simulink model "ASM_Traffic_V2X_Complete_Model_2"  (R2019a)
settings: Solver=ode1  StartTime=SIM.tstart.v  StopTime=Inf  FixedStep=SIM.StepSize.v  RelTol=1e-3
PostLoadFcn:
  | if any(exist('dsrtsu_mdlpostloadfcn', 'file') ~= 0), dsrtsu_mdlpostloadfcn('Execute', bdroot); end
  | try, asm_mdl_postloadfcn(bdroot, 'UpdateModel', 2200); catch, disp(lasterr); end,
undefined symbols (not defined in the file): _SensorPnts_1, _SensorPnts_13, _SensorPnts_17, _SensorPnts_21, _SensorPnts_25, _SensorPnts_29, _SensorPnts_33, _SensorPnts_37, _SensorPnts_41, _SensorPnts_45, _SensorPnts_49, _SensorPnts_5, _SensorPnts_53, _SensorPnts_57, _SensorPnts_9, _to_, CPT, G5A, ITS, MDL, rad, s_to_rpm, SIM
libraries: simulink x169, ASM_VehicleDynamics_lib x126, ASM_Traffic_lib x83, ASM_Utils_lib x49, mdbs x45, ASM_Environment_lib x17, dspindex x12, dsaV2xLibraryAux x10, dsmpblib x6, dsaV2xAsn1Library x4, dsaV2xLibrary x4, ASM_BrakeHydraulics_lib x4
(part 27 of 36)

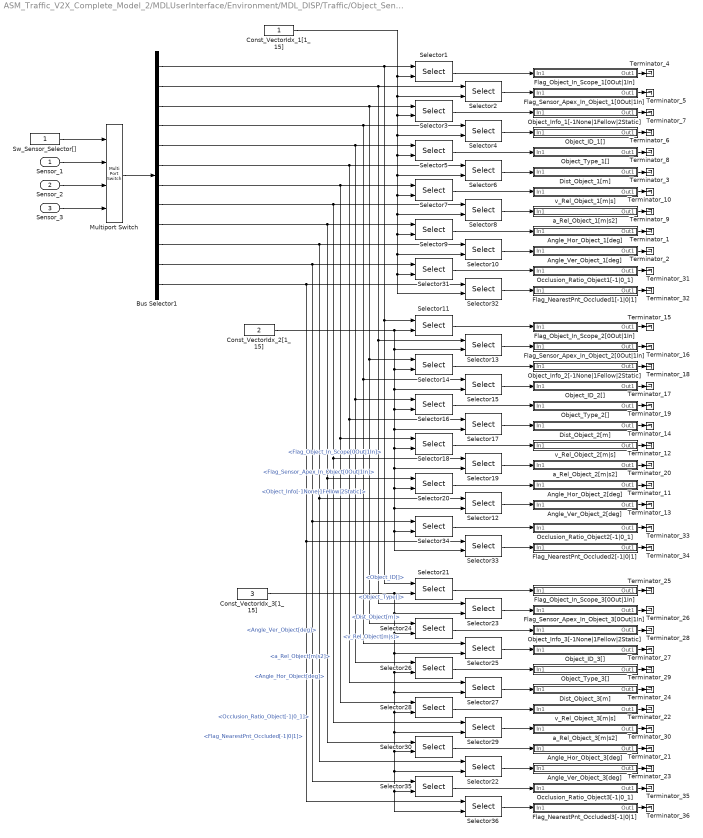
== system ASM_Traffic_V2X_Complete_Model_2/MDLUserInterface/Environment/MDL_DISP/Traffic/Object_Sensor_3D/IdxSelect_3DSensor ==
  Sensor_1 : Inport
  Sensor_2 : Inport  Port=2
  Sensor_3 : Inport  Port=3
  Angle_Hor_Object_1[deg] : Subsystem
      mask Display: disp('')
  Angle_Hor_Object_2[deg] : Subsystem
      mask Display: disp('')
  Angle_Hor_Object_3[deg] : Subsystem
      mask Display: disp('')
  Angle_Ver_Object_1[deg] : Subsystem
      mask Display: disp('')
  Angle_Ver_Object_2[deg] : Subsystem
      mask Display: disp('')
  Angle_Ver_Object_3[deg] : Subsystem
      mask Display: disp('')
  Bus Selector1 : BusSelector  OutputSignals=Info.Flag_Object_In_Scope[0Out|1In],Info.Flag_Sensor_Apex_In_Object[0Out|1In],SensorOutput.Object_Info[-1None|1Fellow|2Static],SensorOutput.Object_ID[],SensorOutput.Object_Type[],SensorOutput.Dist_Object[m],SensorOutput.v_Rel_Object[m|s],SensorOutput.a_Rel_Object[m|s2],SensorOutput.Angle_Hor_Object[deg],SensorOutput.Angle_Ver_Object[deg],SensorOutput.Occlusion_Ratio_Object[-1|0_1],SensorOutput.Flag_NearestPnt_Occluded[-1|0|1]
  Const_VectorIdx_1[1_15] : Constant
  Const_VectorIdx_2[1_15] : Constant  Value=2
  Const_VectorIdx_3[1_15] : Constant  Value=3
  Dist_Object_1[m] : Subsystem
      mask Display: disp('')
  Dist_Object_2[m] : Subsystem
      mask Display: disp('')
  Dist_Object_3[m] : Subsystem
      mask Display: disp('')
  Flag_NearestPnt_Occluded1[-1|0|1] : Subsystem
      mask Display: disp('')
  Flag_NearestPnt_Occluded2[-1|0|1] : Subsystem
      mask Display: disp('')
  Flag_NearestPnt_Occluded3[-1|0|1] : Subsystem
      mask Display: disp('')
  Flag_Object_In_Scope_1[0Out|1In] : Subsystem
      mask Display: disp('')
  Flag_Object_In_Scope_2[0Out|1In] : Subsystem
      mask Display: disp('')
  Flag_Object_In_Scope_3[0Out|1In] : Subsystem
      mask Display: disp('')
  Flag_Sensor_Apex_In_Object_1[0Out|1In] : Subsystem
      mask Display: disp('')
  Flag_Sensor_Apex_In_Object_2[0Out|1In] : Subsystem
      mask Display: disp('')
  Flag_Sensor_Apex_In_Object_3[0Out|1In] : Subsystem
      mask Display: disp('')
  Multiport Switch : MultiPortSwitch
  Object_ID_1[] : Subsystem
      mask Display: disp('')
  Object_ID_2[] : Subsystem
      mask Display: disp('')
  Object_ID_3[] : Subsystem
      mask Display: disp('')
  Object_Info_1[-1None|1Fellow|2Static] : Subsystem
      mask Display: disp('')
  Object_Info_2[-1None|1Fellow|2Static] : Subsystem
      mask Display: disp('')
  Object_Info_3[-1None|1Fellow|2Static] : Subsystem
      mask Display: disp('')
  Object_Type_1[] : Subsystem
      mask Display: disp('')
  Object_Type_2[] : Subsystem
      mask Display: disp('')
  Object_Type_3[] : Subsystem
      mask Display: disp('')
  Occlusion_Ratio_Object1[-1|0_1] : Subsystem
      mask Display: disp('')
  Occlusion_Ratio_Object2[-1|0_1] : Subsystem
      mask Display: disp('')
  Occlusion_Ratio_Object3[-1|0_1] : Subsystem
      mask Display: disp('')
  Selector{1..36} (36 alike) : Selector  InputPortWidth=MDL.Traffic.Sensors.ObjectSensor3D_Calculation.Const_Sensor_Output_Dimension.v  IndexOptions=Index vector (port)  Indices=[1 3]  OutputSizes=1
  Sw_Sensor_Selector[] : Constant
  Terminator_{1..36} (36 alike) : Terminator
  a_Rel_Object_1[m|s2] : Subsystem
      mask Display: disp('')
  a_Rel_Object_2[m|s2] : Subsystem
      mask Display: disp('')
  a_Rel_Object_3[m|s2] : Subsystem
      mask Display: disp('')
  v_Rel_Object_1[m|s] : Subsystem
      mask Display: disp('')
  v_Rel_Object_2[m|s] : Subsystem
      mask Display: disp('')
  v_Rel_Object_3[m|s] : Subsystem
      mask Display: disp('')
  wires:
  Multiport Switch/1 -> Bus Selector1/1
  Sensor_3/1 -> Multiport Switch/4
  Sensor_2/1 -> Multiport Switch/3
  Sensor_1/1 -> Multiport Switch/2
  Sw_Sensor_Selector[]/1 -> Multiport Switch/1
  Const_VectorIdx_3[1_15]/1 -> Selector21/2, Selector23/2, Selector25/2, Selector26/2, Selector27/2, Selector28/2, Selector29/2, Selector30/2, Selector36/2, Selector35/2, Selector22/2, Selector24/2
  Const_VectorIdx_2[1_15]/1 -> Selector11/2, Selector13/2, Selector14/2, Selector15/2, Selector16/2, Selector18/2, Selector19/2, Selector20/2, Selector12/2, Selector33/2, Selector34/2, Selector17/2
  v_Rel_Object_3[m|s]/1(Out1) -> Terminator_22/1
  a_Rel_Object_3[m|s2]/1(Out1) -> Terminator_30/1
  Object_Type_3[]/1(Out1) -> Terminator_29/1
  Object_Info_3[-1None|1Fellow|2Static]/1(Out1) -> Terminator_28/1
  Object_ID_3[]/1(Out1) -> Terminator_27/1
  Flag_Sensor_Apex_In_Object_3[0Out|1In]/1(Out1) -> Terminator_26/1
  Flag_Object_In_Scope_3[0Out|1In]/1(Out1) -> Terminator_25/1
  Dist_Object_3[m]/1(Out1) -> Terminator_24/1
  Angle_Ver_Object_3[deg]/1(Out1) -> Terminator_23/1
  Angle_Hor_Object_3[deg]/1(Out1) -> Terminator_21/1
  Selector22/1 -> Angle_Ver_Object_3[deg]/1(In1)
  Selector30/1 -> Angle_Hor_Object_3[deg]/1(In1)
  Selector29/1 -> a_Rel_Object_3[m|s2]/1(In1)
  Selector28/1 -> v_Rel_Object_3[m|s]/1(In1)
  Selector27/1 -> Dist_Object_3[m]/1(In1)
  Selector26/1 -> Object_Type_3[]/1(In1)
  Selector24/1 -> Object_Info_3[-1None|1Fellow|2Static]/1(In1)
  Selector25/1 -> Object_ID_3[]/1(In1)
  Selector23/1 -> Flag_Sensor_Apex_In_Object_3[0Out|1In]/1(In1)
  Selector21/1 -> Flag_Object_In_Scope_3[0Out|1In]/1(In1)
  v_Rel_Object_2[m|s]/1(Out1) -> Terminator_12/1
  a_Rel_Object_2[m|s2]/1(Out1) -> Terminator_20/1
  Object_Type_2[]/1(Out1) -> Terminator_19/1
  Object_Info_2[-1None|1Fellow|2Static]/1(Out1) -> Terminator_18/1
  Object_ID_2[]/1(Out1) -> Terminator_17/1
  Flag_Sensor_Apex_In_Object_2[0Out|1In]/1(Out1) -> Terminator_16/1
  Flag_Object_In_Scope_2[0Out|1In]/1(Out1) -> Terminator_15/1
  Dist_Object_2[m]/1(Out1) -> Terminator_14/1
  Angle_Ver_Object_2[deg]/1(Out1) -> Terminator_13/1
  Angle_Hor_Object_2[deg]/1(Out1) -> Terminator_11/1
  Selector12/1 -> Angle_Ver_Object_2[deg]/1(In1)
  Selector20/1 -> Angle_Hor_Object_2[deg]/1(In1)
  Selector19/1 -> a_Rel_Object_2[m|s2]/1(In1)
  Selector18/1 -> v_Rel_Object_2[m|s]/1(In1)
  Selector17/1 -> Dist_Object_2[m]/1(In1)
  Selector16/1 -> Object_Type_2[]/1(In1)
  Selector14/1 -> Object_Info_2[-1None|1Fellow|2Static]/1(In1)
  Selector15/1 -> Object_ID_2[]/1(In1)
  Selector13/1 -> Flag_Sensor_Apex_In_Object_2[0Out|1In]/1(In1)
  Selector11/1 -> Flag_Object_In_Scope_2[0Out|1In]/1(In1)
  v_Rel_Object_1[m|s]/1(Out1) -> Terminator_10/1
  a_Rel_Object_1[m|s2]/1(Out1) -> Terminator_9/1
  Object_Type_1[]/1(Out1) -> Terminator_8/1
  Object_Info_1[-1None|1Fellow|2Static]/1(Out1) -> Terminator_7/1
  Object_ID_1[]/1(Out1) -> Terminator_6/1
  Flag_Sensor_Apex_In_Object_1[0Out|1In]/1(Out1) -> Terminator_5/1
  Flag_Object_In_Scope_1[0Out|1In]/1(Out1) -> Terminator_4/1
  Dist_Object_1[m]/1(Out1) -> Terminator_3/1
  Angle_Ver_Object_1[deg]/1(Out1) -> Terminator_2/1
  Angle_Hor_Object_1[deg]/1(Out1) -> Terminator_1/1
  Selector10/1 -> Angle_Ver_Object_1[deg]/1(In1)
  Selector9/1 -> Angle_Hor_Object_1[deg]/1(In1)
  Selector8/1 -> a_Rel_Object_1[m|s2]/1(In1)
  Selector7/1 -> v_Rel_Object_1[m|s]/1(In1)
  Selector6/1 -> Dist_Object_1[m]/1(In1)
  Selector5/1 -> Object_Type_1[]/1(In1)
  Selector3/1 -> Object_Info_1[-1None|1Fellow|2Static]/1(In1)
  Selector4/1 -> Object_ID_1[]/1(In1)
  Selector2/1 -> Flag_Sensor_Apex_In_Object_1[0Out|1In]/1(In1)
  Selector1/1 -> Flag_Object_In_Scope_1[0Out|1In]/1(In1)
  Const_VectorIdx_1[1_15]/1 -> Selector1/2, Selector2/2, Selector31/2, Selector32/2, Selector10/2, Selector9/2, Selector8/2, Selector7/2, Selector6/2, Selector5/2, Selector4/2, Selector3/2
  Bus Selector1/10 -> Selector10/1, Selector22/1, Selector12/1  "<Angle_Ver_Object[deg]>"
  Bus Selector1/9 -> Selector9/1, Selector30/1, Selector20/1  "<Angle_Hor_Object[deg]>"
  Bus Selector1/8 -> Selector8/1, Selector29/1, Selector19/1  "<a_Rel_Object[m|s2]>"
  Bus Selector1/7 -> Selector7/1, Selector28/1, Selector18/1  "<v_Rel_Object[m|s]>"
  Bus Selector1/6 -> Selector6/1, Selector27/1, Selector17/1  "<Dist_Object[m]>"
  Bus Selector1/5 -> Selector5/1, Selector26/1, Selector16/1  "<Object_Type[]>"
  Bus Selector1/4 -> Selector4/1, Selector25/1, Selector15/1  "<Object_ID[]>"
  Bus Selector1/3 -> Selector3/1, Selector24/1, Selector14/1  "<Object_Info[-1None|1Fellow|2Static]>"
  Bus Selector1/2 -> Selector2/1, Selector23/1, Selector13/1  "<Flag_Sensor_Apex_In_Object[0Out|1In]>"
  Bus Selector1/1 -> Selector1/1, Selector21/1, Selector11/1  "<Flag_Object_In_Scope[0Out|1In]>"
  Bus Selector1/11 -> Selector34/1, Selector35/1, Selector31/1  "<Occlusion_Ratio_Object[-1|0_1]>"
  Bus Selector1/12 -> Selector36/1, Selector33/1, Selector32/1  "<Flag_NearestPnt_Occluded[-1|0|1]>"
  Selector31/1 -> Occlusion_Ratio_Object1[-1|0_1]/1(In1)
  Selector32/1 -> Flag_NearestPnt_Occluded1[-1|0|1]/1(In1)
  Occlusion_Ratio_Object1[-1|0_1]/1(Out1) -> Terminator_31/1
  Flag_NearestPnt_Occluded1[-1|0|1]/1(Out1) -> Terminator_32/1
  Selector34/1 -> Occlusion_Ratio_Object2[-1|0_1]/1(In1)
  Selector33/1 -> Flag_NearestPnt_Occluded2[-1|0|1]/1(In1)
  Occlusion_Ratio_Object2[-1|0_1]/1(Out1) -> Terminator_33/1
  Flag_NearestPnt_Occluded2[-1|0|1]/1(Out1) -> Terminator_34/1
  Flag_NearestPnt_Occluded3[-1|0|1]/1(Out1) -> Terminator_36/1
  Occlusion_Ratio_Object3[-1|0_1]/1(Out1) -> Terminator_35/1
  Selector36/1 -> Flag_NearestPnt_Occluded3[-1|0|1]/1(In1)
  Selector35/1 -> Occlusion_Ratio_Object3[-1|0_1]/1(In1)

== system ASM_Traffic_V2X_Complete_Model_2/MDLUserInterface/Environment/MDL_DISP/Traffic/Object_Sensor_3D/IndexConflict_Info[] ==
  In1 : Inport
  Out1 : Outport
  wires:
  In1/1 -> Out1/1

== system ASM_Traffic_V2X_Complete_Model_2/MDLUserInterface/Environment/MDL_DISP/Traffic/Object_Sensor_3D/InputDataSamplePulse[0|1] ==
  In1 : Inport
  Out1 : Outport
  wires:
  In1/1 -> Out1/1

== system ASM_Traffic_V2X_Complete_Model_2/MDLUserInterface/Environment/MDL_DISP/Traffic/Object_Sensor_3D/Object_ID[] ==
  In1 : Inport
  Out1 : Outport
  wires:
  In1/1 -> Out1/1

== system ASM_Traffic_V2X_Complete_Model_2/MDLUserInterface/Environment/MDL_DISP/Traffic/Object_Sensor_3D/Object_ID[]1 ==
  In1 : Inport
  Out1 : Outport
  wires:
  In1/1 -> Out1/1

== system ASM_Traffic_V2X_Complete_Model_2/MDLUserInterface/Environment/MDL_DISP/Traffic/Object_Sensor_3D/Object_ID[]2 ==
  In1 : Inport
  Out1 : Outport
  wires:
  In1/1 -> Out1/1

== system ASM_Traffic_V2X_Complete_Model_2/MDLUserInterface/Environment/MDL_DISP/Traffic/Object_Sensor_3D/Object_Info[-1None|1Fellow|2Static] ==
  In1 : Inport
  Out1 : Outport
  wires:
  In1/1 -> Out1/1

== system ASM_Traffic_V2X_Complete_Model_2/MDLUserInterface/Environment/MDL_DISP/Traffic/Object_Sensor_3D/Object_Info[-1None|1Fellow|2Static]1 ==
  In1 : Inport
  Out1 : Outport
  wires:
  In1/1 -> Out1/1

== system ASM_Traffic_V2X_Complete_Model_2/MDLUserInterface/Environment/MDL_DISP/Traffic/Object_Sensor_3D/Object_Info[-1None|1Fellow|2Static]2 ==
  In1 : Inport
  Out1 : Outport
  wires:
  In1/1 -> Out1/1

== system ASM_Traffic_V2X_Complete_Model_2/MDLUserInterface/Environment/MDL_DISP/Traffic/Object_Sensor_3D/Object_Sensor_3D_VisualizationData ==
  TrafficBus : Inport
  Bus Selector1 : BusSelector  OutputSignals=Sensors.Object_Sensor_3D.Sensor_1_Front_Long,Sensors.Object_Sensor_3D.Sensor_2_Front_Mid,Sensors.Object_Sensor_3D.Sensor_3_Rear
  Bus Selector2 : BusSelector  OutputSignals=Sensors.Object_Sensor_3D.Sensor_1_Front_Long,Sensors.Object_Sensor_3D.Sensor_2_Front_Mid,Sensors.Object_Sensor_3D.Sensor_3_Rear
  Bus Selector9 : BusSelector  OutputSignals=Sensors.Object_Sensor_3D.Sensor_1_Front_Long,Sensors.Object_Sensor_3D.Sensor_2_Front_Mid,Sensors.Object_Sensor_3D.Sensor_3_Rear
  Sensor_1_Front_Long_CustomPoints : Subsystem
  Sensor_1_Front_Long_NearestPoints : Subsystem
  Sensor_1_Front_Long_RadarReflectionPoints : Subsystem
  Sensor_2_Front_Mid_CustomPoints : Subsystem
  Sensor_2_Front_Mid_NearestPoints : Subsystem
  Sensor_2_Front_Mid_RadarReflectionPoints : Subsystem
  Sensor_3_Rear_CustomPoints : Subsystem
  Sensor_3_Rear_NearestPoints : Subsystem
  Sensor_3_Rear_RadarReflectionPoints : Subsystem
  wires:
  Bus Selector9/3 -> Sensor_3_Rear_NearestPoints/1(Sensor)  "<Sensor_3_Rear>"
  Bus Selector9/2 -> Sensor_2_Front_Mid_NearestPoints/1(Sensor)  "<Sensor_2_Front_Mid>"
  TrafficBus/1 -> Bus Selector2/1, Bus Selector1/1, Bus Selector9/1
  Bus Selector9/1 -> Sensor_1_Front_Long_NearestPoints/1(Sensor)  "<Sensor_1_Front_Long>"
  Bus Selector1/1 -> Sensor_1_Front_Long_RadarReflectionPoints/1(Sensor)  "<Sensor_1_Front_Long>"
  Bus Selector1/2 -> Sensor_2_Front_Mid_RadarReflectionPoints/1(Sensor)  "<Sensor_2_Front_Mid>"
  Bus Selector1/3 -> Sensor_3_Rear_RadarReflectionPoints/1(Sensor)  "<Sensor_3_Rear>"
  Bus Selector2/1 -> Sensor_1_Front_Long_CustomPoints/1(Sensor)  "<Sensor_1_Front_Long>"
  Bus Selector2/2 -> Sensor_2_Front_Mid_CustomPoints/1(Sensor)  "<Sensor_2_Front_Mid>"
  Bus Selector2/3 -> Sensor_3_Rear_CustomPoints/1(Sensor)  "<Sensor_3_Rear>"

== system ASM_Traffic_V2X_Complete_Model_2/MDLUserInterface/Environment/MDL_DISP/Traffic/Object_Sensor_3D/Object_Type[] ==
  In1 : Inport
  Out1 : Outport
  wires:
  In1/1 -> Out1/1

== system ASM_Traffic_V2X_Complete_Model_2/MDLUserInterface/Environment/MDL_DISP/Traffic/Object_Sensor_3D/Object_Type[]1 ==
  In1 : Inport
  Out1 : Outport
  wires:
  In1/1 -> Out1/1

== system ASM_Traffic_V2X_Complete_Model_2/MDLUserInterface/Environment/MDL_DISP/Traffic/Object_Sensor_3D/Object_Type[]2 ==
  In1 : Inport
  Out1 : Outport
  wires:
  In1/1 -> Out1/1

== system ASM_Traffic_V2X_Complete_Model_2/MDLUserInterface/Environment/MDL_DISP/Traffic/Object_Sensor_3D/Occlusion_Ratio_Object[-1|0_1] ==
  In1 : Inport
  Out1 : Outport
  wires:
  In1/1 -> Out1/1

== system ASM_Traffic_V2X_Complete_Model_2/MDLUserInterface/Environment/MDL_DISP/Traffic/Object_Sensor_3D/Occlusion_Ratio_Object[-1|0_1]1 ==
  In1 : Inport
  Out1 : Outport
  wires:
  In1/1 -> Out1/1

== system ASM_Traffic_V2X_Complete_Model_2/MDLUserInterface/Environment/MDL_DISP/Traffic/Object_Sensor_3D/Occlusion_Ratio_Object[-1|0_1]2 ==
  In1 : Inport
  Out1 : Outport
  wires:
  In1/1 -> Out1/1

== system ASM_Traffic_V2X_Complete_Model_2/MDLUserInterface/Environment/MDL_DISP/Traffic/Object_Sensor_3D/SensorEnable[0Off|1On] ==
  In1 : Inport
  Out1 : Outport
  wires:
  In1/1 -> Out1/1

== system ASM_Traffic_V2X_Complete_Model_2/MDLUserInterface/Environment/MDL_DISP/Traffic/Object_Sensor_3D/SensorIdx_Selected[] ==
  In1 : Inport
  Out1 : Outport
  wires:
  In1/1 -> Out1/1

== system ASM_Traffic_V2X_Complete_Model_2/MDLUserInterface/Environment/MDL_DISP/Traffic/Object_Sensor_3D/SensorSelection_Data[0|1] ==
  In1 : Inport
  Out1 : Outport
  wires:
  In1/1 -> Out1/1

== system ASM_Traffic_V2X_Complete_Model_2/MDLUserInterface/Environment/MDL_DISP/Traffic/Object_Sensor_3D/a_Rel_Object[m|s2] ==
  In1 : Inport
  Out1 : Outport
  wires:
  In1/1 -> Out1/1

== system ASM_Traffic_V2X_Complete_Model_2/MDLUserInterface/Environment/MDL_DISP/Traffic/Object_Sensor_3D/a_Rel_Object[m|s2]1 ==
  In1 : Inport
  Out1 : Outport
  wires:
  In1/1 -> Out1/1

== system ASM_Traffic_V2X_Complete_Model_2/MDLUserInterface/Environment/MDL_DISP/Traffic/Object_Sensor_3D/a_Rel_Object[m|s2]2 ==
  In1 : Inport
  Out1 : Outport
  wires:
  In1/1 -> Out1/1

== system ASM_Traffic_V2X_Complete_Model_2/MDLUserInterface/Environment/MDL_DISP/Traffic/Object_Sensor_3D/v_Rel_Object[m|s] ==
  In1 : Inport
  Out1 : Outport
  wires:
  In1/1 -> Out1/1

== system ASM_Traffic_V2X_Complete_Model_2/MDLUserInterface/Environment/MDL_DISP/Traffic/Object_Sensor_3D/v_Rel_Object[m|s]1 ==
  In1 : Inport
  Out1 : Outport
  wires:
  In1/1 -> Out1/1

== system ASM_Traffic_V2X_Complete_Model_2/MDLUserInterface/Environment/MDL_DISP/Traffic/Object_Sensor_3D/v_Rel_Object[m|s]2 ==
  In1 : Inport
  Out1 : Outport
  wires:
  In1/1 -> Out1/1

== system ASM_Traffic_V2X_Complete_Model_2/MDLUserInterface/Environment/MDL_DISP/Traffic/Traffic_Sign_Sensor/Angle_CoorSys_E[x;y;z][deg] ==
  In1 : Inport
  Out1 : Outport
  wires:
  In1/1 -> Out1/1

== system ASM_Traffic_V2X_Complete_Model_2/MDLUserInterface/Environment/MDL_DISP/Traffic/Traffic_Sign_Sensor/Angle_Hor_Rel[deg] ==
  In1 : Inport
  Out1 : Outport
  wires:
  In1/1 -> Out1/1

== system ASM_Traffic_V2X_Complete_Model_2/MDLUserInterface/Environment/MDL_DISP/Traffic/Traffic_Sign_Sensor/Angle_Ver_Rel[] ==
  In1 : Inport
  Out1 : Outport
  wires:
  In1/1 -> Out1/1

== system ASM_Traffic_V2X_Complete_Model_2/MDLUserInterface/Environment/MDL_DISP/Traffic/Traffic_Sign_Sensor/Distance[m] ==
  In1 : Inport
  Out1 : Outport
  wires:
  In1/1 -> Out1/1

== system ASM_Traffic_V2X_Complete_Model_2/MDLUserInterface/Environment/MDL_DISP/Traffic/Traffic_Sign_Sensor/GetTrfSgnDataByIndex_1 ==
  SelectSignDataByIndex : Inport
  TrafficBus : Inport  Port=2
  Saturation : Saturate  UpperLimit=MDL.Traffic.Sensors.TrafficSignSensorDyn_Calculation.Const_Sensor_Output_Dimension.v  LowerLimit=1
  SwitchObjectData : Subsystem
  SwitchObjectPosition : Subsystem
  SwitchSignProperties : Subsystem
  Traffic_Sign_Valid[0|1] : Outport
  TrafficObject_ID[] : Outport  Port=2
  TrafficObject_Type[] : Outport  Port=3
  Parent_Object_ID[] : Outport  Port=4
  Pos_CoorSys_E[x;y;z][m] : Outport  Port=5
  Angle_CoorSys_E[x;y;z][deg] : Outport  Port=6
  Pos_CoorSys_S[x;y;z][m] : Outport  Port=7
  Angle_Hor_Rel[deg] : Outport  Port=8
  Angle_Ver_Rel[deg] : Outport  Port=9
  Distance[m] : Outport  Port=10
  Traffic_Sign_Type[] : Outport  Port=11
  Traffic_Sign_Subtype[] : Outport  Port=12
  Traffic_Sign_Value[] : Outport  Port=13
  Traffic_Sign_Country[] : Outport  Port=14
  Traffic_Sign_Visibility[0_100] : Outport  Port=15
  Object_State[] : Outport  Port=16
  Object_Stream_ID[] : Outport  Port=17
  Traffic_Sign_Lanes[] : Outport  Port=18
  wires:
  Saturation/1 -> SwitchSignProperties/2(Switch), SwitchObjectPosition/2(Switch), SwitchObjectData/2(Switch)
  SwitchObjectData/3(TrafficObject_Type[]) -> TrafficObject_Type[]/1
  SelectSignDataByIndex/1 -> Saturation/1
  TrafficBus/1 -> SwitchSignProperties/1(TrafficBus), SwitchObjectPosition/1(TrafficBus), SwitchObjectData/1(TrafficBus)
  SwitchObjectData/2(TrafficObject_ID[]) -> TrafficObject_ID[]/1
  SwitchObjectData/1(Traffic_Sign_Valid[0|1]) -> Traffic_Sign_Valid[0|1]/1
  SwitchObjectData/4(Parent_Object_ID[]) -> Parent_Object_ID[]/1
  SwitchObjectPosition/1(Pos_CoorSys_E[x;y;z][m]) -> Pos_CoorSys_E[x;y;z][m]/1
  SwitchObjectPosition/2(Angle_CoorSys_E[x;y;z][deg]) -> Angle_CoorSys_E[x;y;z][deg]/1
  SwitchObjectPosition/3(Pos_CoorSys_S[x;y;z][m]) -> Pos_CoorSys_S[x;y;z][m]/1
  SwitchObjectPosition/4(Angle_Hor_Rel[deg]) -> Angle_Hor_Rel[deg]/1
  SwitchObjectPosition/5(Angle_Ver_Rel[deg]) -> Angle_Ver_Rel[deg]/1
  SwitchObjectPosition/6(Distance[m]) -> Distance[m]/1
  SwitchSignProperties/1(Traffic_Sign_Type[]) -> Traffic_Sign_Type[]/1
  SwitchSignProperties/2(Traffic_Sign_Subtype[]) -> Traffic_Sign_Subtype[]/1
  SwitchSignProperties/3(Traffic_Sign_Value[]) -> Traffic_Sign_Value[]/1
  SwitchSignProperties/4(Traffic_Sign_Country[]) -> Traffic_Sign_Country[]/1
  SwitchSignProperties/5(Traffic_Sign_Visibility[0_100]) -> Traffic_Sign_Visibility[0_100]/1
  SwitchSignProperties/6(Object_State[]) -> Object_State[]/1
  SwitchSignProperties/7(Object_Stream_ID[]) -> Object_Stream_ID[]/1
  SwitchSignProperties/8(Traffic_Sign_Lanes[]) -> Traffic_Sign_Lanes[]/1

== system ASM_Traffic_V2X_Complete_Model_2/MDLUserInterface/Environment/MDL_DISP/Traffic/Traffic_Sign_Sensor/Object_State[] ==
  In1 : Inport
  Out1 : Outport
  wires:
  In1/1 -> Out1/1

== system ASM_Traffic_V2X_Complete_Model_2/MDLUserInterface/Environment/MDL_DISP/Traffic/Traffic_Sign_Sensor/Object_Stream_ID[] ==
  In1 : Inport
  Out1 : Outport
  wires:
  In1/1 -> Out1/1

== system ASM_Traffic_V2X_Complete_Model_2/MDLUserInterface/Environment/MDL_DISP/Traffic/Traffic_Sign_Sensor/Parent_Object_ID[] ==
  In1 : Inport
  Out1 : Outport
  wires:
  In1/1 -> Out1/1

== system ASM_Traffic_V2X_Complete_Model_2/MDLUserInterface/Environment/MDL_DISP/Traffic/Traffic_Sign_Sensor/Pos_CoorSys_E[x;y;z][m] ==
  In1 : Inport
  Out1 : Outport
  wires:
  In1/1 -> Out1/1

== system ASM_Traffic_V2X_Complete_Model_2/MDLUserInterface/Environment/MDL_DISP/Traffic/Traffic_Sign_Sensor/Pos_CoorSys_S[x;y;z][m] ==
  In1 : Inport
  Out1 : Outport
  wires:
  In1/1 -> Out1/1

== system ASM_Traffic_V2X_Complete_Model_2/MDLUserInterface/Environment/MDL_DISP/Traffic/Traffic_Sign_Sensor/Sign_Valid[0|1] ==
  In1 : Inport
  Out1 : Outport
  wires:
  In1/1 -> Out1/1

== system ASM_Traffic_V2X_Complete_Model_2/MDLUserInterface/Environment/MDL_DISP/Traffic/Traffic_Sign_Sensor/TrafficObject_ID[] ==
  In1 : Inport
  Out1 : Outport
  wires:
  In1/1 -> Out1/1

== system ASM_Traffic_V2X_Complete_Model_2/MDLUserInterface/Environment/MDL_DISP/Traffic/Traffic_Sign_Sensor/TrafficObject_Type[] ==
  In1 : Inport
  Out1 : Outport
  wires:
  In1/1 -> Out1/1

== system ASM_Traffic_V2X_Complete_Model_2/MDLUserInterface/Environment/MDL_DISP/Traffic/Traffic_Sign_Sensor/TrafficSignSensor_Data_Valid[0|1] ==
  In1 : Inport
  Out1 : Outport
  wires:
  In1/1 -> Out1/1

== system ASM_Traffic_V2X_Complete_Model_2/MDLUserInterface/Environment/MDL_DISP/Traffic/Traffic_Sign_Sensor/TrafficSignSensor_Sfcn_State[] ==
  In1 : Inport
  Out1 : Outport
  wires:
  In1/1 -> Out1/1

== system ASM_Traffic_V2X_Complete_Model_2/MDLUserInterface/Environment/MDL_DISP/Traffic/Traffic_Sign_Sensor/Traffic_Sign_Country[] ==
  In1 : Inport
  Out1 : Outport
  wires:
  In1/1 -> Out1/1

== system ASM_Traffic_V2X_Complete_Model_2/MDLUserInterface/Environment/MDL_DISP/Traffic/Traffic_Sign_Sensor/Traffic_Sign_Lanes[] ==
  In1 : Inport
  Out1 : Outport
  wires:
  In1/1 -> Out1/1

== system ASM_Traffic_V2X_Complete_Model_2/MDLUserInterface/Environment/MDL_DISP/Traffic/Traffic_Sign_Sensor/Traffic_Sign_Subtype[] ==
  In1 : Inport
  Out1 : Outport
  wires:
  In1/1 -> Out1/1

== system ASM_Traffic_V2X_Complete_Model_2/MDLUserInterface/Environment/MDL_DISP/Traffic/Traffic_Sign_Sensor/Traffic_Sign_Type[] ==
  In1 : Inport
  Out1 : Outport
  wires:
  In1/1 -> Out1/1

== system ASM_Traffic_V2X_Complete_Model_2/MDLUserInterface/Environment/MDL_DISP/Traffic/Traffic_Sign_Sensor/Traffic_Sign_Value[] ==
  In1 : Inport
  Out1 : Outport
  wires:
  In1/1 -> Out1/1

== system ASM_Traffic_V2X_Complete_Model_2/MDLUserInterface/Environment/MDL_DISP/Traffic/Traffic_Sign_Sensor/Traffic_Sign_Visibility[0_100] ==
  In1 : Inport
  Out1 : Outport
  wires:
  In1/1 -> Out1/1

== system ASM_Traffic_V2X_Complete_Model_2/MDLUserInterface/MotionDeskInterface/MOTION_DESK_INTERFACE/Coding_Fellows/Coding1/SwitchDelay ==
  Turnlight_L : Inport
  Turnlight_R : Inport  Port=2
  Add : Sum
  Compare To Constant : simulink/Logic and Bit Operations/Compare To Constant  relop=>  const=2  OutDataTypeStr=boolean
  Logical Operator1 : Logic  AllPortsSameDT=off  OutDataTypeStr=boolean
  Logical Operator2 : Logic  AllPortsSameDT=off  OutDataTypeStr=boolean
  Logical Operator4 : Logic  AllPortsSameDT=off  OutDataTypeStr=boolean
  Relational Operator3 : RelationalOperator  Operator=>  OutDataTypeStr=boolean  RndMeth=Nearest
  Switch : Switch  Criteria=u2 > Threshold
  Unit Delay{1..3,6} (4 alike) : UnitDelay  SampleTime=-1
  one : Constant  OutDataTypeStr=uint32
  zero : Constant  Value=0  OutDataTypeStr=uint32
  Turnlight_L_out : Outport
  Turnlight_R_out : Outport  Port=2
  wires:
  Unit Delay6/1 -> Logical Operator4/1
  Unit Delay3/1 -> Logical Operator2/1
  Unit Delay2/1 -> Relational Operator3/2
  Logical Operator1/1 -> Relational Operator3/1, Unit Delay2/1
  Relational Operator3/1 -> Switch/2
  zero/1 -> Switch/1
  Switch/1 -> Unit Delay1/1
  one/1 -> Add/1
  Unit Delay1/1 -> Add/2, Compare To Constant/1
  Add/1 -> Switch/3
  Compare To Constant/1 -> Logical Operator2/2, Logical Operator4/2
  Logical Operator2/1 -> Turnlight_L_out/1
  Logical Operator4/1 -> Turnlight_R_out/1
  Turnlight_L/1 -> Unit Delay3/1, Logical Operator1/1
  Turnlight_R/1 -> Unit Delay6/1, Logical Operator1/2

== system ASM_Traffic_V2X_Complete_Model_2/MDLUserInterface/MotionDeskInterface/MOTION_DESK_INTERFACE/Coding_Fellows/Coding10/SwitchDelay ==
  Turnlight_L : Inport
  Turnlight_R : Inport  Port=2
  Add : Sum
  Compare To Constant : simulink/Logic and Bit Operations/Compare To Constant  relop=>  const=2  OutDataTypeStr=boolean
  Logical Operator1 : Logic  AllPortsSameDT=off  OutDataTypeStr=boolean
  Logical Operator2 : Logic  AllPortsSameDT=off  OutDataTypeStr=boolean
  Logical Operator4 : Logic  AllPortsSameDT=off  OutDataTypeStr=boolean
  Relational Operator3 : RelationalOperator  Operator=>  OutDataTypeStr=boolean  RndMeth=Nearest
  Switch : Switch  Criteria=u2 > Threshold
  Unit Delay{1..3,6} (4 alike) : UnitDelay  SampleTime=-1
  one : Constant  OutDataTypeStr=uint32
  zero : Constant  Value=0  OutDataTypeStr=uint32
  Turnlight_L_out : Outport
  Turnlight_R_out : Outport  Port=2
  wires:
  Turnlight_R/1 -> Logical Operator1/2, Unit Delay6/1
  Turnlight_L/1 -> Logical Operator1/1, Unit Delay3/1
  Logical Operator4/1 -> Turnlight_R_out/1
  Logical Operator2/1 -> Turnlight_L_out/1
  Compare To Constant/1 -> Logical Operator4/2, Logical Operator2/2
  Add/1 -> Switch/3
  Unit Delay1/1 -> Compare To Constant/1, Add/2
  one/1 -> Add/1
  Switch/1 -> Unit Delay1/1
  zero/1 -> Switch/1
  Relational Operator3/1 -> Switch/2
  Logical Operator1/1 -> Unit Delay2/1, Relational Operator3/1
  Unit Delay2/1 -> Relational Operator3/2
  Unit Delay3/1 -> Logical Operator2/1
  Unit Delay6/1 -> Logical Operator4/1

== system ASM_Traffic_V2X_Complete_Model_2/MDLUserInterface/MotionDeskInterface/MOTION_DESK_INTERFACE/Coding_Fellows/Coding11/SwitchDelay ==
  Turnlight_L : Inport
  Turnlight_R : Inport  Port=2
  Add : Sum
  Compare To Constant : simulink/Logic and Bit Operations/Compare To Constant  relop=>  const=2  OutDataTypeStr=boolean
  Logical Operator1 : Logic  AllPortsSameDT=off  OutDataTypeStr=boolean
  Logical Operator2 : Logic  AllPortsSameDT=off  OutDataTypeStr=boolean
  Logical Operator4 : Logic  AllPortsSameDT=off  OutDataTypeStr=boolean
  Relational Operator3 : RelationalOperator  Operator=>  OutDataTypeStr=boolean  RndMeth=Nearest
  Switch : Switch  Criteria=u2 > Threshold
  Unit Delay{1..3,6} (4 alike) : UnitDelay  SampleTime=-1
  one : Constant  OutDataTypeStr=uint32
  zero : Constant  Value=0  OutDataTypeStr=uint32
  Turnlight_L_out : Outport
  Turnlight_R_out : Outport  Port=2
  wires:
  Unit Delay6/1 -> Logical Operator4/1
  Unit Delay3/1 -> Logical Operator2/1
  Unit Delay2/1 -> Relational Operator3/2
  Logical Operator1/1 -> Relational Operator3/1, Unit Delay2/1
  Relational Operator3/1 -> Switch/2
  zero/1 -> Switch/1
  Switch/1 -> Unit Delay1/1
  one/1 -> Add/1
  Unit Delay1/1 -> Add/2, Compare To Constant/1
  Add/1 -> Switch/3
  Compare To Constant/1 -> Logical Operator2/2, Logical Operator4/2
  Logical Operator2/1 -> Turnlight_L_out/1
  Logical Operator4/1 -> Turnlight_R_out/1
  Turnlight_L/1 -> Unit Delay3/1, Logical Operator1/1
  Turnlight_R/1 -> Unit Delay6/1, Logical Operator1/2

== system ASM_Traffic_V2X_Complete_Model_2/MDLUserInterface/MotionDeskInterface/MOTION_DESK_INTERFACE/Coding_Fellows/Coding12/SwitchDelay ==
  Turnlight_L : Inport
  Turnlight_R : Inport  Port=2
  Add : Sum
  Compare To Constant : simulink/Logic and Bit Operations/Compare To Constant  relop=>  const=2  OutDataTypeStr=boolean
  Logical Operator1 : Logic  AllPortsSameDT=off  OutDataTypeStr=boolean
  Logical Operator2 : Logic  AllPortsSameDT=off  OutDataTypeStr=boolean
  Logical Operator4 : Logic  AllPortsSameDT=off  OutDataTypeStr=boolean
  Relational Operator3 : RelationalOperator  Operator=>  OutDataTypeStr=boolean  RndMeth=Nearest
  Switch : Switch  Criteria=u2 > Threshold
  Unit Delay{1..3,6} (4 alike) : UnitDelay  SampleTime=-1
  one : Constant  OutDataTypeStr=uint32
  zero : Constant  Value=0  OutDataTypeStr=uint32
  Turnlight_L_out : Outport
  Turnlight_R_out : Outport  Port=2
  wires:
  Turnlight_R/1 -> Logical Operator1/2, Unit Delay6/1
  Turnlight_L/1 -> Logical Operator1/1, Unit Delay3/1
  Logical Operator4/1 -> Turnlight_R_out/1
  Logical Operator2/1 -> Turnlight_L_out/1
  Compare To Constant/1 -> Logical Operator4/2, Logical Operator2/2
  Add/1 -> Switch/3
  Unit Delay1/1 -> Compare To Constant/1, Add/2
  one/1 -> Add/1
  Switch/1 -> Unit Delay1/1
  zero/1 -> Switch/1
  Relational Operator3/1 -> Switch/2
  Logical Operator1/1 -> Unit Delay2/1, Relational Operator3/1
  Unit Delay2/1 -> Relational Operator3/2
  Unit Delay3/1 -> Logical Operator2/1
  Unit Delay6/1 -> Logical Operator4/1

== system ASM_Traffic_V2X_Complete_Model_2/MDLUserInterface/MotionDeskInterface/MOTION_DESK_INTERFACE/Coding_Fellows/Coding13/SwitchDelay ==
  Turnlight_L : Inport
  Turnlight_R : Inport  Port=2
  Add : Sum
  Compare To Constant : simulink/Logic and Bit Operations/Compare To Constant  relop=>  const=2  OutDataTypeStr=boolean
  Logical Operator1 : Logic  AllPortsSameDT=off  OutDataTypeStr=boolean
  Logical Operator2 : Logic  AllPortsSameDT=off  OutDataTypeStr=boolean
  Logical Operator4 : Logic  AllPortsSameDT=off  OutDataTypeStr=boolean
  Relational Operator3 : RelationalOperator  Operator=>  OutDataTypeStr=boolean  RndMeth=Nearest
  Switch : Switch  Criteria=u2 > Threshold
  Unit Delay{1..3,6} (4 alike) : UnitDelay  SampleTime=-1
  one : Constant  OutDataTypeStr=uint32
  zero : Constant  Value=0  OutDataTypeStr=uint32
  Turnlight_L_out : Outport
  Turnlight_R_out : Outport  Port=2
  wires:
  Unit Delay6/1 -> Logical Operator4/1
  Unit Delay3/1 -> Logical Operator2/1
  Unit Delay2/1 -> Relational Operator3/2
  Logical Operator1/1 -> Relational Operator3/1, Unit Delay2/1
  Relational Operator3/1 -> Switch/2
  zero/1 -> Switch/1
  Switch/1 -> Unit Delay1/1
  one/1 -> Add/1
  Unit Delay1/1 -> Add/2, Compare To Constant/1
  Add/1 -> Switch/3
  Compare To Constant/1 -> Logical Operator2/2, Logical Operator4/2
  Logical Operator2/1 -> Turnlight_L_out/1
  Logical Operator4/1 -> Turnlight_R_out/1
  Turnlight_L/1 -> Unit Delay3/1, Logical Operator1/1
  Turnlight_R/1 -> Unit Delay6/1, Logical Operator1/2

== system ASM_Traffic_V2X_Complete_Model_2/MDLUserInterface/MotionDeskInterface/MOTION_DESK_INTERFACE/Coding_Fellows/Coding14/SwitchDelay ==
  Turnlight_L : Inport
  Turnlight_R : Inport  Port=2
  Add : Sum
  Compare To Constant : simulink/Logic and Bit Operations/Compare To Constant  relop=>  const=2  OutDataTypeStr=boolean
  Logical Operator1 : Logic  AllPortsSameDT=off  OutDataTypeStr=boolean
  Logical Operator2 : Logic  AllPortsSameDT=off  OutDataTypeStr=boolean
  Logical Operator4 : Logic  AllPortsSameDT=off  OutDataTypeStr=boolean
  Relational Operator3 : RelationalOperator  Operator=>  OutDataTypeStr=boolean  RndMeth=Nearest
  Switch : Switch  Criteria=u2 > Threshold
  Unit Delay{1..3,6} (4 alike) : UnitDelay  SampleTime=-1
  one : Constant  OutDataTypeStr=uint32
  zero : Constant  Value=0  OutDataTypeStr=uint32
  Turnlight_L_out : Outport
  Turnlight_R_out : Outport  Port=2
  wires:
  Turnlight_R/1 -> Logical Operator1/2, Unit Delay6/1
  Turnlight_L/1 -> Logical Operator1/1, Unit Delay3/1
  Logical Operator4/1 -> Turnlight_R_out/1
  Logical Operator2/1 -> Turnlight_L_out/1
  Compare To Constant/1 -> Logical Operator4/2, Logical Operator2/2
  Add/1 -> Switch/3
  Unit Delay1/1 -> Compare To Constant/1, Add/2
  one/1 -> Add/1
  Switch/1 -> Unit Delay1/1
  zero/1 -> Switch/1
  Relational Operator3/1 -> Switch/2
  Logical Operator1/1 -> Unit Delay2/1, Relational Operator3/1
  Unit Delay2/1 -> Relational Operator3/2
  Unit Delay3/1 -> Logical Operator2/1
  Unit Delay6/1 -> Logical Operator4/1

== system ASM_Traffic_V2X_Complete_Model_2/MDLUserInterface/MotionDeskInterface/MOTION_DESK_INTERFACE/Coding_Fellows/Coding15/SwitchDelay ==
  Turnlight_L : Inport
  Turnlight_R : Inport  Port=2
  Add : Sum
  Compare To Constant : simulink/Logic and Bit Operations/Compare To Constant  relop=>  const=2  OutDataTypeStr=boolean
  Logical Operator1 : Logic  AllPortsSameDT=off  OutDataTypeStr=boolean
  Logical Operator2 : Logic  AllPortsSameDT=off  OutDataTypeStr=boolean
  Logical Operator4 : Logic  AllPortsSameDT=off  OutDataTypeStr=boolean
  Relational Operator3 : RelationalOperator  Operator=>  OutDataTypeStr=boolean  RndMeth=Nearest
  Switch : Switch  Criteria=u2 > Threshold
  Unit Delay{1..3,6} (4 alike) : UnitDelay  SampleTime=-1
  one : Constant  OutDataTypeStr=uint32
  zero : Constant  Value=0  OutDataTypeStr=uint32
  Turnlight_L_out : Outport
  Turnlight_R_out : Outport  Port=2
  wires:
  Unit Delay6/1 -> Logical Operator4/1
  Unit Delay3/1 -> Logical Operator2/1
  Unit Delay2/1 -> Relational Operator3/2
  Logical Operator1/1 -> Relational Operator3/1, Unit Delay2/1
  Relational Operator3/1 -> Switch/2
  zero/1 -> Switch/1
  Switch/1 -> Unit Delay1/1
  one/1 -> Add/1
  Unit Delay1/1 -> Add/2, Compare To Constant/1
  Add/1 -> Switch/3
  Compare To Constant/1 -> Logical Operator2/2, Logical Operator4/2
  Logical Operator2/1 -> Turnlight_L_out/1
  Logical Operator4/1 -> Turnlight_R_out/1
  Turnlight_L/1 -> Unit Delay3/1, Logical Operator1/1
  Turnlight_R/1 -> Unit Delay6/1, Logical Operator1/2

== system ASM_Traffic_V2X_Complete_Model_2/MDLUserInterface/MotionDeskInterface/MOTION_DESK_INTERFACE/Coding_Fellows/Coding2/SwitchDelay ==
  Turnlight_L : Inport
  Turnlight_R : Inport  Port=2
  Add : Sum
  Compare To Constant : simulink/Logic and Bit Operations/Compare To Constant  relop=>  const=2  OutDataTypeStr=boolean
  Logical Operator1 : Logic  AllPortsSameDT=off  OutDataTypeStr=boolean
  Logical Operator2 : Logic  AllPortsSameDT=off  OutDataTypeStr=boolean
  Logical Operator4 : Logic  AllPortsSameDT=off  OutDataTypeStr=boolean
  Relational Operator3 : RelationalOperator  Operator=>  OutDataTypeStr=boolean  RndMeth=Nearest
  Switch : Switch  Criteria=u2 > Threshold
  Unit Delay{1..3,6} (4 alike) : UnitDelay  SampleTime=-1
  one : Constant  OutDataTypeStr=uint32
  zero : Constant  Value=0  OutDataTypeStr=uint32
  Turnlight_L_out : Outport
  Turnlight_R_out : Outport  Port=2
  wires:
  Turnlight_R/1 -> Logical Operator1/2, Unit Delay6/1
  Turnlight_L/1 -> Logical Operator1/1, Unit Delay3/1
  Logical Operator4/1 -> Turnlight_R_out/1
  Logical Operator2/1 -> Turnlight_L_out/1
  Compare To Constant/1 -> Logical Operator4/2, Logical Operator2/2
  Add/1 -> Switch/3
  Unit Delay1/1 -> Compare To Constant/1, Add/2
  one/1 -> Add/1
  Switch/1 -> Unit Delay1/1
  zero/1 -> Switch/1
  Relational Operator3/1 -> Switch/2
  Logical Operator1/1 -> Unit Delay2/1, Relational Operator3/1
  Unit Delay2/1 -> Relational Operator3/2
  Unit Delay3/1 -> Logical Operator2/1
  Unit Delay6/1 -> Logical Operator4/1

== system ASM_Traffic_V2X_Complete_Model_2/MDLUserInterface/MotionDeskInterface/MOTION_DESK_INTERFACE/Coding_Fellows/Coding3/SwitchDelay ==
  Turnlight_L : Inport
  Turnlight_R : Inport  Port=2
  Add : Sum
  Compare To Constant : simulink/Logic and Bit Operations/Compare To Constant  relop=>  const=2  OutDataTypeStr=boolean
  Logical Operator1 : Logic  AllPortsSameDT=off  OutDataTypeStr=boolean
  Logical Operator2 : Logic  AllPortsSameDT=off  OutDataTypeStr=boolean
  Logical Operator4 : Logic  AllPortsSameDT=off  OutDataTypeStr=boolean
  Relational Operator3 : RelationalOperator  Operator=>  OutDataTypeStr=boolean  RndMeth=Nearest
  Switch : Switch  Criteria=u2 > Threshold
  Unit Delay{1..3,6} (4 alike) : UnitDelay  SampleTime=-1
  one : Constant  OutDataTypeStr=uint32
  zero : Constant  Value=0  OutDataTypeStr=uint32
  Turnlight_L_out : Outport
  Turnlight_R_out : Outport  Port=2
  wires:
  Unit Delay6/1 -> Logical Operator4/1
  Unit Delay3/1 -> Logical Operator2/1
  Unit Delay2/1 -> Relational Operator3/2
  Logical Operator1/1 -> Relational Operator3/1, Unit Delay2/1
  Relational Operator3/1 -> Switch/2
  zero/1 -> Switch/1
  Switch/1 -> Unit Delay1/1
  one/1 -> Add/1
  Unit Delay1/1 -> Add/2, Compare To Constant/1
  Add/1 -> Switch/3
  Compare To Constant/1 -> Logical Operator2/2, Logical Operator4/2
  Logical Operator2/1 -> Turnlight_L_out/1
  Logical Operator4/1 -> Turnlight_R_out/1
  Turnlight_L/1 -> Unit Delay3/1, Logical Operator1/1
  Turnlight_R/1 -> Unit Delay6/1, Logical Operator1/2

== system ASM_Traffic_V2X_Complete_Model_2/MDLUserInterface/MotionDeskInterface/MOTION_DESK_INTERFACE/Coding_Fellows/Coding4/SwitchDelay ==
  Turnlight_L : Inport
  Turnlight_R : Inport  Port=2
  Add : Sum
  Compare To Constant : simulink/Logic and Bit Operations/Compare To Constant  relop=>  const=2  OutDataTypeStr=boolean
  Logical Operator1 : Logic  AllPortsSameDT=off  OutDataTypeStr=boolean
  Logical Operator2 : Logic  AllPortsSameDT=off  OutDataTypeStr=boolean
  Logical Operator4 : Logic  AllPortsSameDT=off  OutDataTypeStr=boolean
  Relational Operator3 : RelationalOperator  Operator=>  OutDataTypeStr=boolean  RndMeth=Nearest
  Switch : Switch  Criteria=u2 > Threshold
  Unit Delay{1..3,6} (4 alike) : UnitDelay  SampleTime=-1
  one : Constant  OutDataTypeStr=uint32
  zero : Constant  Value=0  OutDataTypeStr=uint32
  Turnlight_L_out : Outport
  Turnlight_R_out : Outport  Port=2
  wires:
  Turnlight_R/1 -> Logical Operator1/2, Unit Delay6/1
  Turnlight_L/1 -> Logical Operator1/1, Unit Delay3/1
  Logical Operator4/1 -> Turnlight_R_out/1
  Logical Operator2/1 -> Turnlight_L_out/1
  Compare To Constant/1 -> Logical Operator4/2, Logical Operator2/2
  Add/1 -> Switch/3
  Unit Delay1/1 -> Compare To Constant/1, Add/2
  one/1 -> Add/1
  Switch/1 -> Unit Delay1/1
  zero/1 -> Switch/1
  Relational Operator3/1 -> Switch/2
  Logical Operator1/1 -> Unit Delay2/1, Relational Operator3/1
  Unit Delay2/1 -> Relational Operator3/2
  Unit Delay3/1 -> Logical Operator2/1
  Unit Delay6/1 -> Logical Operator4/1

== system ASM_Traffic_V2X_Complete_Model_2/MDLUserInterface/MotionDeskInterface/MOTION_DESK_INTERFACE/Coding_Fellows/Coding5/SwitchDelay ==
  Turnlight_L : Inport
  Turnlight_R : Inport  Port=2
  Add : Sum
  Compare To Constant : simulink/Logic and Bit Operations/Compare To Constant  relop=>  const=2  OutDataTypeStr=boolean
  Logical Operator1 : Logic  AllPortsSameDT=off  OutDataTypeStr=boolean
  Logical Operator2 : Logic  AllPortsSameDT=off  OutDataTypeStr=boolean
  Logical Operator4 : Logic  AllPortsSameDT=off  OutDataTypeStr=boolean
  Relational Operator3 : RelationalOperator  Operator=>  OutDataTypeStr=boolean  RndMeth=Nearest
  Switch : Switch  Criteria=u2 > Threshold
  Unit Delay{1..3,6} (4 alike) : UnitDelay  SampleTime=-1
  one : Constant  OutDataTypeStr=uint32
  zero : Constant  Value=0  OutDataTypeStr=uint32
  Turnlight_L_out : Outport
  Turnlight_R_out : Outport  Port=2
  wires:
  Unit Delay6/1 -> Logical Operator4/1
  Unit Delay3/1 -> Logical Operator2/1
  Unit Delay2/1 -> Relational Operator3/2
  Logical Operator1/1 -> Relational Operator3/1, Unit Delay2/1
  Relational Operator3/1 -> Switch/2
  zero/1 -> Switch/1
  Switch/1 -> Unit Delay1/1
  one/1 -> Add/1
  Unit Delay1/1 -> Add/2, Compare To Constant/1
  Add/1 -> Switch/3
  Compare To Constant/1 -> Logical Operator2/2, Logical Operator4/2
  Logical Operator2/1 -> Turnlight_L_out/1
  Logical Operator4/1 -> Turnlight_R_out/1
  Turnlight_L/1 -> Unit Delay3/1, Logical Operator1/1
  Turnlight_R/1 -> Unit Delay6/1, Logical Operator1/2

== system ASM_Traffic_V2X_Complete_Model_2/MDLUserInterface/MotionDeskInterface/MOTION_DESK_INTERFACE/Coding_Fellows/Coding6/SwitchDelay ==
  Turnlight_L : Inport
  Turnlight_R : Inport  Port=2
  Add : Sum
  Compare To Constant : simulink/Logic and Bit Operations/Compare To Constant  relop=>  const=2  OutDataTypeStr=boolean
  Logical Operator1 : Logic  AllPortsSameDT=off  OutDataTypeStr=boolean
  Logical Operator2 : Logic  AllPortsSameDT=off  OutDataTypeStr=boolean
  Logical Operator4 : Logic  AllPortsSameDT=off  OutDataTypeStr=boolean
  Relational Operator3 : RelationalOperator  Operator=>  OutDataTypeStr=boolean  RndMeth=Nearest
  Switch : Switch  Criteria=u2 > Threshold
  Unit Delay{1..3,6} (4 alike) : UnitDelay  SampleTime=-1
  one : Constant  OutDataTypeStr=uint32
  zero : Constant  Value=0  OutDataTypeStr=uint32
  Turnlight_L_out : Outport
  Turnlight_R_out : Outport  Port=2
  wires:
  Turnlight_R/1 -> Logical Operator1/2, Unit Delay6/1
  Turnlight_L/1 -> Logical Operator1/1, Unit Delay3/1
  Logical Operator4/1 -> Turnlight_R_out/1
  Logical Operator2/1 -> Turnlight_L_out/1
  Compare To Constant/1 -> Logical Operator4/2, Logical Operator2/2
  Add/1 -> Switch/3
  Unit Delay1/1 -> Compare To Constant/1, Add/2
  one/1 -> Add/1
  Switch/1 -> Unit Delay1/1
  zero/1 -> Switch/1
  Relational Operator3/1 -> Switch/2
  Logical Operator1/1 -> Unit Delay2/1, Relational Operator3/1
  Unit Delay2/1 -> Relational Operator3/2
  Unit Delay3/1 -> Logical Operator2/1
  Unit Delay6/1 -> Logical Operator4/1

== system ASM_Traffic_V2X_Complete_Model_2/MDLUserInterface/MotionDeskInterface/MOTION_DESK_INTERFACE/Coding_Fellows/Coding7/SwitchDelay ==
  Turnlight_L : Inport
  Turnlight_R : Inport  Port=2
  Add : Sum
  Compare To Constant : simulink/Logic and Bit Operations/Compare To Constant  relop=>  const=2  OutDataTypeStr=boolean
  Logical Operator1 : Logic  AllPortsSameDT=off  OutDataTypeStr=boolean
  Logical Operator2 : Logic  AllPortsSameDT=off  OutDataTypeStr=boolean
  Logical Operator4 : Logic  AllPortsSameDT=off  OutDataTypeStr=boolean
  Relational Operator3 : RelationalOperator  Operator=>  OutDataTypeStr=boolean  RndMeth=Nearest
  Switch : Switch  Criteria=u2 > Threshold
  Unit Delay{1..3,6} (4 alike) : UnitDelay  SampleTime=-1
  one : Constant  OutDataTypeStr=uint32
  zero : Constant  Value=0  OutDataTypeStr=uint32
  Turnlight_L_out : Outport
  Turnlight_R_out : Outport  Port=2
  wires:
  Unit Delay6/1 -> Logical Operator4/1
  Unit Delay3/1 -> Logical Operator2/1
  Unit Delay2/1 -> Relational Operator3/2
  Logical Operator1/1 -> Relational Operator3/1, Unit Delay2/1
  Relational Operator3/1 -> Switch/2
  zero/1 -> Switch/1
  Switch/1 -> Unit Delay1/1
  one/1 -> Add/1
  Unit Delay1/1 -> Add/2, Compare To Constant/1
  Add/1 -> Switch/3
  Compare To Constant/1 -> Logical Operator2/2, Logical Operator4/2
  Logical Operator2/1 -> Turnlight_L_out/1
  Logical Operator4/1 -> Turnlight_R_out/1
  Turnlight_L/1 -> Unit Delay3/1, Logical Operator1/1
  Turnlight_R/1 -> Unit Delay6/1, Logical Operator1/2

== system ASM_Traffic_V2X_Complete_Model_2/MDLUserInterface/MotionDeskInterface/MOTION_DESK_INTERFACE/Coding_Fellows/Coding8/SwitchDelay ==
  Turnlight_L : Inport
  Turnlight_R : Inport  Port=2
  Add : Sum
  Compare To Constant : simulink/Logic and Bit Operations/Compare To Constant  relop=>  const=2  OutDataTypeStr=boolean
  Logical Operator1 : Logic  AllPortsSameDT=off  OutDataTypeStr=boolean
  Logical Operator2 : Logic  AllPortsSameDT=off  OutDataTypeStr=boolean
  Logical Operator4 : Logic  AllPortsSameDT=off  OutDataTypeStr=boolean
  Relational Operator3 : RelationalOperator  Operator=>  OutDataTypeStr=boolean  RndMeth=Nearest
  Switch : Switch  Criteria=u2 > Threshold
  Unit Delay{1..3,6} (4 alike) : UnitDelay  SampleTime=-1
  one : Constant  OutDataTypeStr=uint32
  zero : Constant  Value=0  OutDataTypeStr=uint32
  Turnlight_L_out : Outport
  Turnlight_R_out : Outport  Port=2
  wires:
  Turnlight_R/1 -> Logical Operator1/2, Unit Delay6/1
  Turnlight_L/1 -> Logical Operator1/1, Unit Delay3/1
  Logical Operator4/1 -> Turnlight_R_out/1
  Logical Operator2/1 -> Turnlight_L_out/1
  Compare To Constant/1 -> Logical Operator4/2, Logical Operator2/2
  Add/1 -> Switch/3
  Unit Delay1/1 -> Compare To Constant/1, Add/2
  one/1 -> Add/1
  Switch/1 -> Unit Delay1/1
  zero/1 -> Switch/1
  Relational Operator3/1 -> Switch/2
  Logical Operator1/1 -> Unit Delay2/1, Relational Operator3/1
  Unit Delay2/1 -> Relational Operator3/2
  Unit Delay3/1 -> Logical Operator2/1
  Unit Delay6/1 -> Logical Operator4/1

== system ASM_Traffic_V2X_Complete_Model_2/MDLUserInterface/MotionDeskInterface/MOTION_DESK_INTERFACE/Coding_Fellows/Coding9/SwitchDelay ==
  Turnlight_L : Inport
  Turnlight_R : Inport  Port=2
  Add : Sum
  Compare To Constant : simulink/Logic and Bit Operations/Compare To Constant  relop=>  const=2  OutDataTypeStr=boolean
  Logical Operator1 : Logic  AllPortsSameDT=off  OutDataTypeStr=boolean
  Logical Operator2 : Logic  AllPortsSameDT=off  OutDataTypeStr=boolean
  Logical Operator4 : Logic  AllPortsSameDT=off  OutDataTypeStr=boolean
  Relational Operator3 : RelationalOperator  Operator=>  OutDataTypeStr=boolean  RndMeth=Nearest
  Switch : Switch  Criteria=u2 > Threshold
  Unit Delay{1..3,6} (4 alike) : UnitDelay  SampleTime=-1
  one : Constant  OutDataTypeStr=uint32
  zero : Constant  Value=0  OutDataTypeStr=uint32
  Turnlight_L_out : Outport
  Turnlight_R_out : Outport  Port=2
  wires:
  Unit Delay6/1 -> Logical Operator4/1
  Unit Delay3/1 -> Logical Operator2/1
  Unit Delay2/1 -> Relational Operator3/2
  Logical Operator1/1 -> Relational Operator3/1, Unit Delay2/1
  Relational Operator3/1 -> Switch/2
  zero/1 -> Switch/1
  Switch/1 -> Unit Delay1/1
  one/1 -> Add/1
  Unit Delay1/1 -> Add/2, Compare To Constant/1
  Add/1 -> Switch/3
  Compare To Constant/1 -> Logical Operator2/2, Logical Operator4/2
  Logical Operator2/1 -> Turnlight_L_out/1
  Logical Operator4/1 -> Turnlight_R_out/1
  Turnlight_L/1 -> Unit Delay3/1, Logical Operator1/1
  Turnlight_R/1 -> Unit Delay6/1, Logical Operator1/2

== system ASM_Traffic_V2X_Complete_Model_2/MDLUserInterface/MotionDeskInterface/MOTION_DESK_INTERFACE/Traffic_Animation/Fellows_Animation/Fellow_1 ==
  Transform_In : Inport
  Pos_x_Fellows[m] : Inport  Port=2
  Pos_y_Fellows[m] : Inport  Port=3
  Pos_z_Fellows[m] : Inport  Port=4
  Angle_Roll_Fellows[deg] : Inport  Port=5
  Angle_Pitch_Fellows[deg] : Inport  Port=6
  Angle_Yaw_Fellows[deg] : Inport  Port=7
  Flag_FellowUsed : Inport  Port=8
  Constant : Constant
  MD_Object : mdbs/MD_Object  strObjId=8  strObjName=Fellow_01  strBlockType=OBJ  bGUIEventOK=0
      settings: SourceProductName=dSPACE MotionDesk Blockset
  Mux : Mux  Inputs=3
  Mux1 : Mux  Inputs=3
  Mux3 : Mux  Inputs=3
  Selector{1..7} (7 alike) : Selector  InputPortWidth=MDL.Traffic.MaxNumFellows.v  IndexOptions=Index vector (port)  Indices=[1 3]  OutputSizes=1
  Terminator : Terminator
  wires:
  Selector4/1 -> Mux1/3
  Selector7/1 -> Mux1/1
  Selector5/1 -> Mux1/2
  MD_Object/1 -> Terminator/1
  Selector6/1 -> Mux3/1, Mux3/3, Mux3/2
  Mux1/1 -> MD_Object/3
  Mux/1 -> MD_Object/2
  Transform_In/1 -> MD_Object/1
  Mux3/1 -> MD_Object/4
  Flag_FellowUsed/1 -> Selector6/1
  Constant/1 -> Selector3/2, Selector4/2, Selector6/2, Selector7/2, Selector5/2, Selector2/2, Selector1/2
  Selector1/1 -> Mux/1
  Selector2/1 -> Mux/2
  Selector3/1 -> Mux/3
  Angle_Yaw_Fellows[deg]/1 -> Selector7/1
  Angle_Pitch_Fellows[deg]/1 -> Selector5/1
  Angle_Roll_Fellows[deg]/1 -> Selector4/1
  Pos_z_Fellows[m]/1 -> Selector3/1
  Pos_y_Fellows[m]/1 -> Selector2/1
  Pos_x_Fellows[m]/1 -> Selector1/1

== system ASM_Traffic_V2X_Complete_Model_2/MDLUserInterface/MotionDeskInterface/MOTION_DESK_INTERFACE/Traffic_Animation/Fellows_Animation/Fellow_10 ==
  Transform_In : Inport
  Pos_x_Fellows[m] : Inport  Port=2
  Pos_y_Fellows[m] : Inport  Port=3
  Pos_z_Fellows[m] : Inport  Port=4
  Angle_Roll_Fellows[deg] : Inport  Port=5
  Angle_Pitch_Fellows[deg] : Inport  Port=6
  Angle_Yaw_Fellows[deg] : Inport  Port=7
  Flag_FellowUsed : Inport  Port=8
  Constant : Constant  Value=10
  MD_Object : mdbs/MD_Object  strObjId=17  strObjName=Fellow_10  strBlockType=OBJ  bGUIEventOK=0
      settings: SourceProductName=dSPACE MotionDesk Blockset
  Mux : Mux  Inputs=3
  Mux1 : Mux  Inputs=3
  Mux3 : Mux  Inputs=3
  Selector{1..7} (7 alike) : Selector  InputPortWidth=MDL.Traffic.MaxNumFellows.v  IndexOptions=Index vector (port)  Indices=[1 3]  OutputSizes=1
  Terminator : Terminator
  wires:
  Pos_x_Fellows[m]/1 -> Selector1/1
  Pos_y_Fellows[m]/1 -> Selector2/1
  Pos_z_Fellows[m]/1 -> Selector3/1
  Angle_Roll_Fellows[deg]/1 -> Selector4/1
  Angle_Pitch_Fellows[deg]/1 -> Selector5/1
  Angle_Yaw_Fellows[deg]/1 -> Selector7/1
  Selector3/1 -> Mux/3
  Selector2/1 -> Mux/2
  Selector1/1 -> Mux/1
  Constant/1 -> Selector1/2, Selector6/2, Selector7/2, Selector5/2, Selector4/2, Selector3/2, Selector2/2
  Flag_FellowUsed/1 -> Selector6/1
  Mux1/1 -> MD_Object/3
  Mux3/1 -> MD_Object/4
  Transform_In/1 -> MD_Object/1
  Mux/1 -> MD_Object/2
  Selector6/1 -> Mux3/2, Mux3/3, Mux3/1
  MD_Object/1 -> Terminator/1
  Selector5/1 -> Mux1/2
  Selector7/1 -> Mux1/1
  Selector4/1 -> Mux1/3
